simulink model "BodyModel_Simulink_OpenLoop"  (R2021a)
settings: Solver=ode23tb  StartTime=0.0  StopTime=20  RelTol=1e-3
undefined symbols (not defined in the file): QuadrotorBodyModel_Object
libraries: uavutilslib x1
settings Model: OrderedModelArguments=off  Creator=prenk  LastModifiedBy=renkert2
settings SolverCC: AlgebraicLoopSolver=TrustRegion
settings DebuggingCC: SFMachineParentedDataDiag=warning

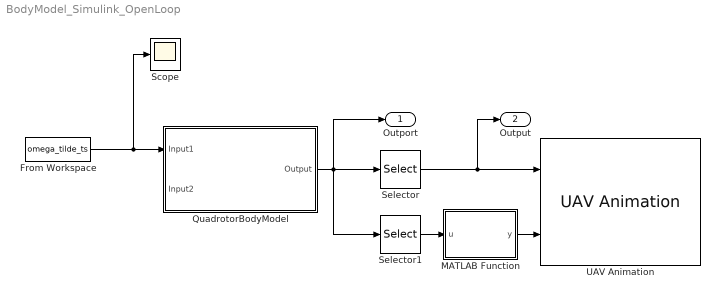
== system BodyModel_Simulink_OpenLoop ==
  From Workspace : FromWorkspace  VariableName=omega_tilde_ts  OutputAfterFinalValue=Holding final value
  MATLAB Function : MATLAB Function  TreatAsAtomicUnit=on
  QuadrotorBodyModel : Subsystem  mask{x_0=QuadrotorBodyModel_Object.x0}
  Scope : Scope
  Selector : Selector  InputPortWidth=QuadrotorBodyModel_Object.Nx  IndexOptions=Index vector (dialog)  Indices=QuadrotorBodyModel_Object.I.x.p  OutputSizes=1
  Selector1 : Selector  InputPortWidth=QuadrotorBodyModel_Object.Nx  IndexOptions=Index vector (dialog)  Indices=QuadrotorBodyModel_Object.I.x.Theta  OutputSizes=1
  UAV Animation : uavutilslib/UAV Animation  UAVType=Multirotor  UAVSize=1  InertialZDirection=Down  SampleTime=-1
      settings: SourceProductBaseCode=UV
  Outport : Outport  SignalName=y_out
  Output : Outport  Port=2  SignalName=p_out
  wires:
  MATLAB Function/1(y) -> UAV Animation/2
  Selector1/1 -> MATLAB Function/1(u)
  Selector/1 -> Output/1, UAV Animation/1
  QuadrotorBodyModel/1(Output) -> Selector1/1, Outport/1, Selector/1
  From Workspace/1 -> Scope/1, QuadrotorBodyModel/1(Input1)

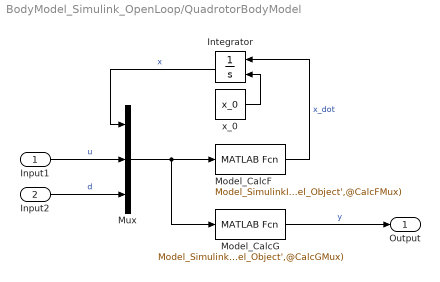
== system BodyModel_Simulink_OpenLoop/QuadrotorBodyModel ==
  Input1 : Inport  PortDimensions=[QuadrotorBodyModel_Object.Nu,1]
  Input2 : Inport  Port=2  PortDimensions=[QuadrotorBodyModel_Object.Nd,1]
  Integrator : Integrator  InitialConditionSource=external
  Model_CalcF : MATLABFcn  MATLABFcn=Model_SimulinkInterpretedFunction(u,'BodyModel_Simulink_OpenLoop','QuadrotorBodyModel_Object',@CalcFMux)  OutputDimensions=QuadrotorBodyModel_Object.Nx
  Model_CalcG : MATLABFcn  MATLABFcn=Model_SimulinkInterpretedFunction(u,'BodyModel_Simulink_OpenLoop','QuadrotorBodyModel_Object',@CalcGMux)  OutputDimensions=QuadrotorBodyModel_Object.Ny
  Mux : Mux  Inputs=3
  x_0 : Constant  Value=x_0  VectorParams1D=off
  Output : Outport
  wires:
  Model_CalcF/1 -> Integrator/1  "x_dot"
  Input1/1 -> Mux/2  "u"
  Model_CalcG/1 -> Output/1  "y"
  x_0/1 -> Integrator/2
  Input2/1 -> Mux/3  "d"
  Integrator/1 -> Mux/1  "x"
  Mux/1 -> Model_CalcG/1, Model_CalcF/1

== matlab function BodyModel_Simulink_OpenLoop/MATLAB Function ==
  data: u input; y output
function y = eul2quatMF(u)
    y = eul2quat([1 -1 1].*fliplr(u'),'ZYX');
end
